simulink model "Dynamics2"  (R2021a)
settings: Solver=VariableStepAuto  StartTime=0.0  StopTime=5  RelTol=1e-3
undefined symbols (not defined in the file): Kc, Kr
settings Model: Creator=Mechatronics  LastModifiedBy=Sizamkele Ngqwemla

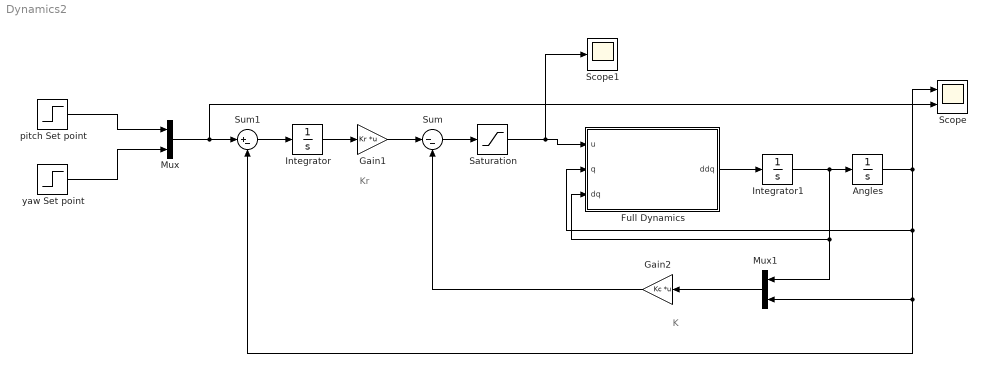
== system Dynamics2 ==
  note: Kr
  note: K
  Angles : Integrator  InitialCondition=[0,0]  ContinuousStateAttributes='angles'
  Full Dynamics : MATLAB Function  TreatAsAtomicUnit=on
  Gain1 : Gain  Gain=Kr  Multiplication=Matrix(K*u)
  Gain2 : Gain  Gain=Kc  Multiplication=Matrix(K*u)
  Integrator : Integrator
  Integrator1 : Integrator  InitialCondition=[0;0]
  Mux : Mux  Inputs=2
  Mux1 : Mux  Inputs=2
  Saturation : Saturate  UpperLimit=24  LowerLimit=-24
  Scope : Scope  NumInputPorts=2
  Scope1 : Scope
  Sum : Sum  Inputs=|--
  Sum1 : Sum  Inputs=|+-
  pitch Set point : Step  Time=0  After=pi/6  SampleTime=0
  yaw Set point : Step  Time=0  After=pi/2  SampleTime=0
  wires:
  pitch Set point/1 -> Mux/1
  yaw Set point/1 -> Mux/2
  Gain1/1 -> Sum/1
  Gain2/1 -> Sum/2
  Integrator/1 -> Gain1/1
  Angles/1 -> Scope/1, Full Dynamics/2(q), Mux1/2, Sum1/2
  Mux1/1 -> Gain2/1
  Mux/1 -> Scope/2, Sum1/1
  Sum1/1 -> Integrator/1
  Integrator1/1 -> Angles/1, Mux1/1, Full Dynamics/3(dq)
  Full Dynamics/1(ddq) -> Integrator1/1
  Sum/1 -> Saturation/1
  Saturation/1 -> Scope1/1, Full Dynamics/1(u)

== matlab function Dynamics2/Full Dynamics ==
  data: ddq output; u input size=[2 1]; q input; dq input
function ddq = fcn(u, q, dq)

Vp = u(1);
Vy = u(2);

tht = q(1);
dtht = dq(1);
dpsil = dq(2);

ddth = (5*Vp)/73 + (20*Vy)/219 - (226*dtht)/219 - (125*tht)/73;
ddpsil = (2*Vy)/11 - (17*Vp)/220 - (211*dpsil)/220;

ddq = [ddth;ddpsil];
